simulink model "RngMod_TrqCalc"  (R2016b)
settings: configuration reference "CodeGenConfigSet" (kept outside this file)
values from neighbouring files (symbols this model uses):
  TRQ_ZERO = fi(0,Trq_Nm)    [init_RngMod_TrqCalc.m]
settings Model: Creator=Wollf  LastModifiedBy=Wollf
settings ConfigSetRef: SourceLocation=Base Workspace

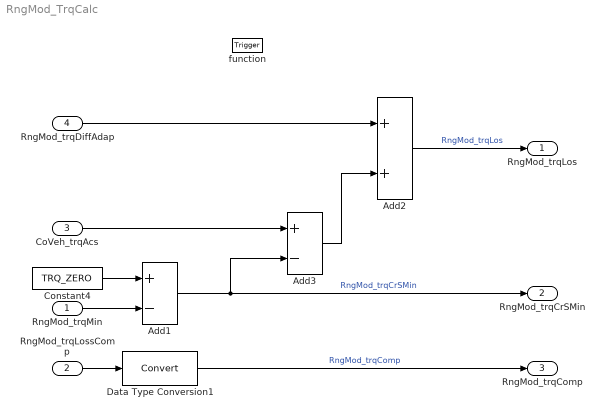
== system RngMod_TrqCalc ==
  RngMod_trqMin : Inport  Tag=Nm  Description=Drag torque (minimum torque)  OutMin=-3276.8  OutMax=3276.7  OutDataTypeStr=Trq_Nm
  RngMod_trqLossComp : Inport  Tag=Nm  Description=compensation for torque  Port=2  OutMin=-3276.8  OutMax=3276.7  OutDataTypeStr=Trq_Nm
  CoVeh_trqAcs : Inport  Tag=Nm  Description=message for demand of accessories  Port=3  OutMin=-3276.8  OutMax=3276.7  OutDataTypeStr=Trq_Nm
  RngMod_trqDiffAdap : Inport  Tag=Nm  Description=Adapted difference torque loss  Port=4  OutMin=-3276.8  OutMax=3276.7  OutDataTypeStr=Trq_Nm
  function : TriggerPort  TriggerType=function-call  VariantControl=Variant
  Add1 : Sum  Inputs=+-  OutDataTypeStr=Inherit: Inherit via back propagation  SaturateOnIntegerOverflow=on  InputSameDT=on
  Add2 : Sum  OutDataTypeStr=Inherit: Inherit via back propagation  SaturateOnIntegerOverflow=on  InputSameDT=on
  Add3 : Sum  Inputs=+-  OutDataTypeStr=Inherit: Inherit via back propagation  SaturateOnIntegerOverflow=on  InputSameDT=on
  Constant4 : Constant  Value=TRQ_ZERO  OutDataTypeStr=Inherit: Inherit via back propagation
  Data Type Conversion1 : DataTypeConversion
  RngMod_trqLos : Outport  Tag=Nm  Description=sum of all engine losses including frictional torque adaption  OutMin=-3276.8  OutMax=3276.7  OutDataTypeStr=Trq_Nm
  RngMod_trqCrSMin : Outport  Tag=Nm  Description=minimal crankshaft torque  Port=2  OutMin=-3276.8  OutMax=3276.7  OutDataTypeStr=Trq_Nm
  RngMod_trqComp : Outport  Tag=Nm  Description=torque to be compensated  Port=3  OutMin=-3276.8  OutMax=3276.7  OutDataTypeStr=Trq_Nm
  wires:
  Constant4/1 -> Add1/1
  Add1/1 -> RngMod_trqCrSMin/1, Add3/2  "RngMod_trqCrSMin"
  Data Type Conversion1/1 -> RngMod_trqComp/1  "RngMod_trqComp"
  RngMod_trqMin/1 -> Add1/2
  RngMod_trqLossComp/1 -> Data Type Conversion1/1
  Add3/1 -> Add2/2
  RngMod_trqDiffAdap/1 -> Add2/1
  Add2/1 -> RngMod_trqLos/1  "RngMod_trqLos"
  CoVeh_trqAcs/1 -> Add3/1
